simulink model "LOG_DATI_GPS_BMP_07_13_provacostanti"  (R2020b)
settings: Solver=ode4  StartTime=0.0  StopTime=Inf  FixedStep=0.02  RelTol=1e-3  EnableMultiTasking=on
PostLoadFcn:
  | , if any(exist('dsrtsu_mdlpostloadfcn', 'file') == [2, 3, 6]), try dsrtsu_mdlpostloadfcn('Execute', bdroot); catch fprintf('Error in PostLoadFcn (dsrtsu_mdlpostloadfcn) for model "%s":\n %s\n', bdroot, lasterr); end, end,
InitFcn:
  | , if any(exist('rtifpga_mdlclblib', 'file') ~= 0), rtifpga_mdlclblib('Init', bdroot); end,
values from neighbouring files (symbols this model uses):
  t_AP = 0.02    [AVVIO_YAK_DATA.m]
libraries: arduinolib x21, simulink_extras x6, svdutilitieslib x2, simulink x2
(part 1 of 3)
Description:
  | Standard RTI1006 template.
  | Supported MATLAB version:  R2020b.
settings Model: Tag=RTI1006  DSRTSU_INTERNAL_RTI_VER=570  DSRTSU_INTERNAL_RTI_TYPE=rti1006  RTICANMMDATA=struct('GeneralSetupData',struct('modelroot','C:\SUBTEAMS_2020_2021\SOFTWARE\AUTOPILOTA\drive1\Load_hardware\Arduino_v2_1','generalsettings',struct('filesettings',struct('destfolder',struct('Name','RTICANMM_FILES','Check',1),'buildfolder',struct('Name','.','Check',1),'AbsDestfolder',struct('Name','C:\SUBTEAMS_2020_2021\SOFTWARE\AUTOPILOTA\drive1\Load_hardware\Arduino_v2_1\RTICANMM_FILES'),'AbsBuildfolder',struct('Name','C:\SUBTEAMS_2020_2021\SOFTWARE\AUTOPILOTA\drive1\Load_hardware\Arduino_v2_1'))),'options',struct('addpaths',1,'rmpaths',1,'addtrcexclusion',true,'cannavigator',struct('checkmonitoring',0),'show_usrtrc',0,'use_usrtrc',0),'advanced',struct('options',ones(1,100)),'MPSetup',{{}},'RTI',struct('Type','ERT','Ver','','Date',''),'modelname','LOG_DATI_GPS_BMP_07_13_provacostanti','block','LOG_DATI_GPS_BMP_07_13_provacostanti'))  DSRTSU_INTERNAL_RTIFPGA=170  SILPILModeSetting=veronly  ExtModeTrigDuration=2  Creator=lapis-dspace  LastModifiedBy=lapis-dspace
settings DataIOCC: ReturnWorkspaceOutputs=off
settings OptimizationCC: BlockReduction=off  EnhancedBackFolding=on  PassReuseOutputArgsAs=Individual arguments  ZeroExternalMemoryAtStartup=off  ZeroInternalMemoryAtStartup=off  MaxStackSize=64  OptimizeBlockOrder=speed  DifferentSizesBufferReuse=on  OptimizationCustomize=off  EfficientTunableParamExpr=on
settings DebuggingCC: ParameterTunabilityLossMsg=error  PregeneratedLibrarySubsystemCodeDiagnostic=none  ArithmeticOperatorsInVariantConditions=warning
settings HardwareCC: ProdBitPerPointer=32  ProdBitPerSizeT=32  ProdBitPerPtrDiffT=32  ProdLargestAtomicInteger=Long  ProdLargestAtomicFloat=Double  ProdWordSize=32  ProdHWDeviceType=ARM Compatible->ARM Cortex  TargetIntDivRoundTo=Zero  TargetEndianess=LittleEndian  TargetHWDeviceType=Custom Processor->Custom
settings ModelReferenceCC: EnableParallelModelReferenceBuilds=on  ParallelModelReferenceMATLABWorkerInit=Load Top Model
settings SFSimCC: SimUseLocalCustomCode=off  MATLABDynamicMemAlloc=off  CustomCodeUndefinedFunction=UseInterfaceOnly
settings RTWCC: Description=Embedded Coder  SystemTargetFile=ert.tlc  HardwareBoard=Arduino Due  TemplateMakefile=ert_default_tmf  RTWUseLocalCustomCode=off  Toolchain=Arduino ARM  BuildConfiguration=Faster Runs
settings CodeAppCC: ForceParamTrailComments=on  IgnoreCustomStorageClasses=off  OperatorAnnotations=on  SimulinkDataObjDesc=on  SFDataObjDesc=on  InsertBlockDesc=on
settings ERTTargetCC: SupportContinuousTime=on  SupportVariableSizeSignals=on  ExtModeTransport=3  ExtModeStaticAllocSize=24576  ExtModeMexFile=ext_xcp  ExtModeIntrfLevel=Level2 - Open
settings ConfigComp: CovMetricSettings=dswe

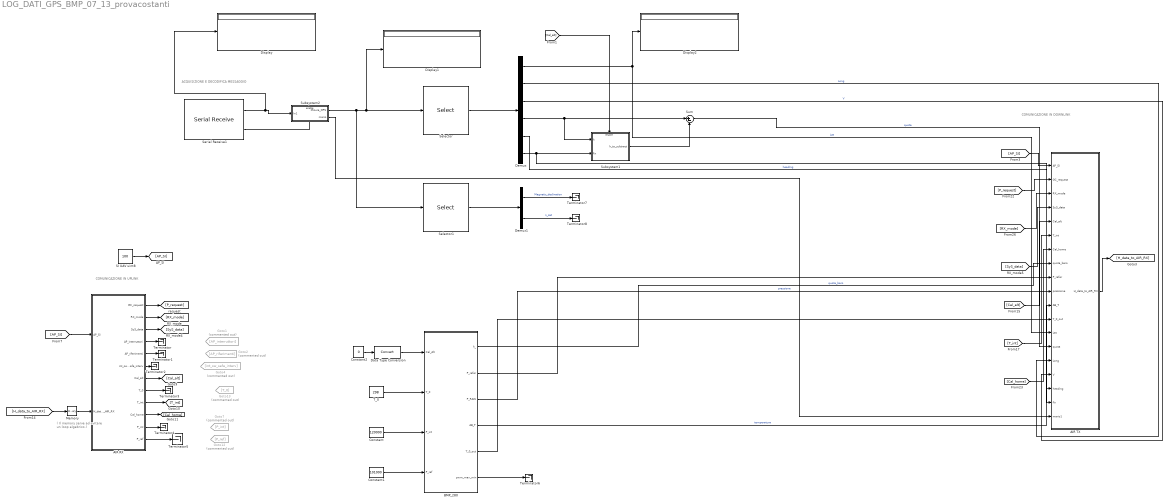
== system LOG_DATI_GPS_BMP_07_13_provacostanti ==
  note: ( Il memory serve ad evitare
      | un loop algebrico.)
  note: COMUNICAZIONE IN UPLINK
  note: COMUNICAZIONE IN DOWNLINK
  note: ACQUISIZIONE E DECODIFICA MESSAGGIO
  AIR RX : Subsystem
  AIR TX : Subsystem
  BMP_280 : Subsystem
  Constant : Constant  Value=120000
  Constant1 : Constant  Value=101000
  Constant2 : Constant  Value=0
  Data Type Conversion : DataTypeConversion
  Demux : Demux  Outputs=6
  Demux1 : Demux  Outputs=2
  Display : Display
  Display1 : Display
  Display2 : Display
  Goto1 : Goto  Commented=on  GotoTag=AP_interruttori
  Goto12 : Goto  Commented=on  GotoTag=P_ref
  Goto13 : Goto  Commented=on  GotoTag=T_0
  Goto2 : Goto  Commented=on  GotoTag=AP_riferimenti
  Goto4 : Goto  Commented=on  GotoTag=int_sw_safe_interv
  Goto7 : Goto  Commented=on  GotoTag=P_int
  Memory : Memory
  SI UAV uint8 : Constant  Value=100  OutDataTypeStr=uint8
  Selector : Selector  InputPortWidth=9  IndexOptions=Index vector (dialog)  Indices=[1 2 3 8 5 6]  OutputSizes=1
  Selector1 : Selector  InputPortWidth=9  IndexOptions=Index vector (dialog)  Indices=[4 7]  OutputSizes=1
  Serial Receive1 : arduinolib/Serial Receive  isARMArch=on  portNumber=1  DataType=uint8  Datalength=32  SampleTime=0.02  showOutStatus=on  blockPlatform=arduino
      settings: SourceProductBaseCode=ARDUINO
  Subsystem1 : Subsystem
  Subsystem2 : Subsystem
  Sum : Sum  Inputs=|+-
  T_0 : Constant  Value=298
  Terminator{,1..8} (9 alike) : Terminator
  wires:
  Constant/1 -> BMP_280/3(P_int)
  BMP_280/1(h_) -> AIR TX/8(quota_baro)  "quota_baro"
  T_0/1 -> BMP_280/2(T_0)
  BMP_280/3(P_RAW) -> AIR TX/10(pressione)  "pressione"
  BMP_280/5(T_0_out) -> AIR TX/12(T_0_out)
  BMP_280/2(P_refer) -> AIR TX/9(P_refer)
  BMP_280/6("pwm_max_min ") -> Terminator6/1
  Constant1/1 -> BMP_280/4(P_ref)
  Constant2/1 -> Data Type Conversion/1
  Data Type Conversion/1 -> BMP_280/1(Cal_Alt)
  AIR RX/9(T_int) -> [T_int]
  AIR RX/10(Cal_home) -> [Cal_home]
  AIR RX/8(T_0) -> Terminator3/1
  AIR RX/6(int_sw_safe_interv) -> Terminator2/1
  AIR RX/1(GC_request) -> [P_request]
  [AP_SI] -> AIR RX/1(AP_SI)
  AIR RX/12(P_ref) -> Terminator5/1
  [SyS_data] -> AIR TX/4(SyS_data)
  [Cal_home] -> AIR TX/7(Cal_home)
  [RX_mode] -> AIR TX/3(RX_mode)
  AIR RX/4(AP_interruttori) -> Terminator/1
  AIR RX/11(P_int) -> Terminator4/1
  [T_int] -> AIR TX/6(T_int)
  [H_data_to_AIR_RX] -> Memory/1
  AIR RX/5(AP_riferimenti) -> Terminator1/1
  [Cal_alt] -> AIR TX/5(Cal_alt)
  [P_request] -> AIR TX/2(GC_request)
  AIR RX/2(RX_mode) -> [RX_mode]
  Memory/1 -> AIR RX/2(H_data_to_AIR_RX)
  SI UAV uint8/1 -> [AP_SI]
  AIR RX/7(Cal_alt) -> [Cal_alt]
  AIR RX/3(SyS_data) -> [SyS_data]
  AIR TX/1(H_data_to_AIR_RX) -> [H_data_to_AIR_RX]
  [AP_SI] -> AIR TX/1(AP_SI)
  BMP_280/4(AB_T) -> AIR TX/11(AB_T)  "temperatura"
  Subsystem2/1(Misure_GPS) -> Selector1/1, Display1/1, Selector/1
  Demux/2 -> AIR TX/15(Long)  "Long"
  Demux1/1 -> Terminator7/1  "Magnetic_declination"
  Demux/6 -> AIR TX/18("fix "), Subsystem1/2(fix)
  Selector/1 -> Demux/1
  [Cal_alt] -> Subsystem1/Enable
  Demux/4 -> Sum/1, Subsystem1/1(h)
  Serial Receive1/1 -> Display/1, Subsystem2/1(In1)
  Demux1/2 -> Terminator8/1  "n_sat"
  Selector1/1 -> Demux1/1
  Demux/5 -> AIR TX/17(heading)  "heading"
  Demux/3 -> AIR TX/16(V)  "V"
  Demux/1 -> Display2/1, AIR TX/13(Lat)  "Lat"
  Sum/1 -> AIR TX/14(quota)  "quota"
  Subsystem2/2(mario) -> AIR TX/19(mario1)
  Subsystem1/1(h_to_subtract) -> Sum/2
  Serial Receive1/2 -> Subsystem2/Enable

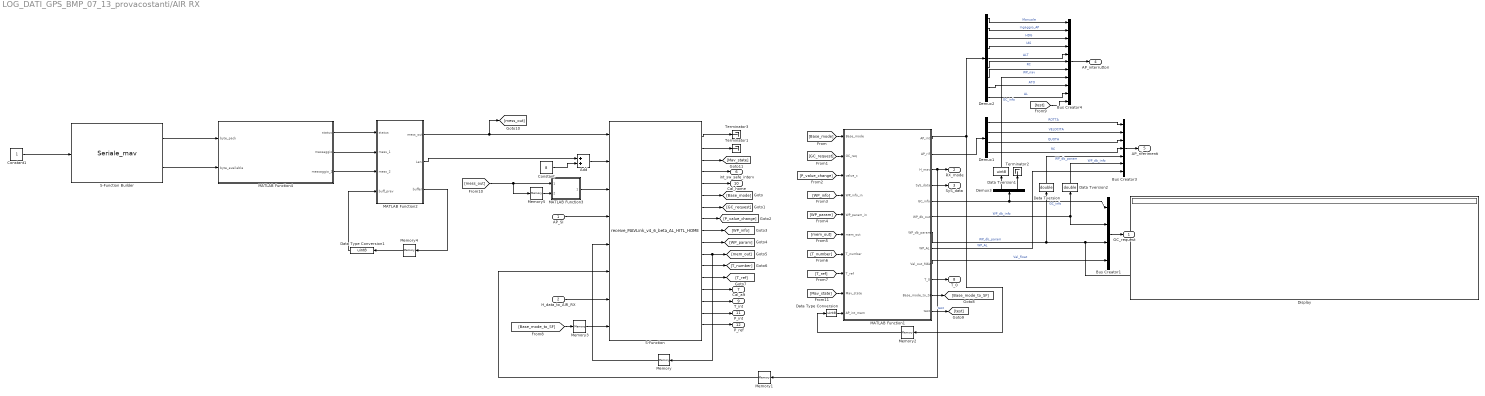
== system LOG_DATI_GPS_BMP_07_13_provacostanti/AIR RX ==
  AP_SI : Inport
  H_data_to_AIR_RX : Inport  Port=2
  Add : Sum  AccumDataTypeStr=int32
  Bus Creator1 : BusCreator  Inputs=4
  Bus Creator3 : BusCreator  Inputs=7
  Bus Creator4 : BusCreator  Inputs=11
  Constant : Constant  Value=8  OutDataTypeStr=int32  SampleTime=-1
  Constant1 : Constant  OutDataTypeStr=uint8
  Data Tversion : DataTypeConversion  OutDataTypeStr=double
  Data Tversion1 : DataTypeConversion  OutDataTypeStr=uint8
  Data Tversion2 : DataTypeConversion  OutDataTypeStr=double
  Data Type Conversion : DataTypeConversion  OutDataTypeStr=uint8
  Data Type Conversion1 : DataTypeConversion  OutDataTypeStr=uint8
  Demux1 : Demux
  Demux2 : Demux  Outputs=9
  Demux3 : Demux  Outputs=[1 2]
  Display : Display
      settings: Floating=on
  MATLAB Function1 : MATLAB Function  TreatAsAtomicUnit=on
  MATLAB Function2 : MATLAB Function  TreatAsAtomicUnit=on
  MATLAB Function3 : MATLAB Function  TreatAsAtomicUnit=on
  MATLAB Function4 : MATLAB Function  TreatAsAtomicUnit=on
  Memory : Memory  InheritSampleTime=on
  Memory1 : Memory  InheritSampleTime=on
  Memory2 : Memory  InitialCondition=[0 0 0 0 0 0 0 0 0]
  Memory3 : Memory
  Memory4 : Memory  InitialCondition=uint8(zeros(3,100))  InheritSampleTime=on
  Memory5 : Memory  InheritSampleTime=on
  S-Function : S-Function  FunctionName=receive_MAVLink_v4_6_beta_AL_HITL_HOME  SFunctionModules='receive_MAVLink_v4_6_beta_AL_HITL_HOME_wrapper'  SFunctionDeploymentMode=off  EnableBusSupport=off
  S-Function Builder : S-Function  InitFcn=try, set_param(gcb,'FunctionName','Seriale_mav'), end  FunctionName=Seriale_mav  SFunctionModules=Seriale_mav_wrapper  SFunctionDeploymentMode=off  EnableBusSupport=off  mask(S-Function Builder){}
      mask help: Simulink:masks:SFunctionBuilder_MD
      mask init:
      | val = [[.9  0.75 0.75 1 1 .9 .9 1]',[1 1 0.75 0.75 .9 .9 1 .9]'];try , sys = get_param(gcb,'SfunBuilderFcnName');if isempty(sys), sys = get_param(gcb,'FunctionName'); end,catch, sys = get_param(gcb,'FunctionName'); end
      settings: CopyFcn=set_param(gcbh,'LinkStatus','none')  PreSaveFcn=try, set_param(gcb,'FunctionName','Seriale_mav'), end  OpenFcn=sfunctionwizard(gcbh)
      mask Display: plot(val(:,1),val(:,2)),disp(sys),port_label('input',1,'inutile'),port_label('output',1,'Messaggio'),port_label('output',2,'serial_available')
  Terminator1 : Terminator
  Terminator2 : Terminator
  Terminator3 : Terminator
  GC_request : Outport  VectorParamsAs1DForOutWhenUnconnected=off
  RX_mode : Outport  Port=2  VectorParamsAs1DForOutWhenUnconnected=off
  SyS_data : Outport  Port=3  VectorParamsAs1DForOutWhenUnconnected=off
  AP_interruttori : Outport  Port=4  VectorParamsAs1DForOutWhenUnconnected=off
  AP_riferimenti : Outport  Port=5  VectorParamsAs1DForOutWhenUnconnected=off
  int_sw_safe_interv : Outport  Port=6  VectorParamsAs1DForOutWhenUnconnected=off
  Cal_alt : Outport  Port=7  VectorParamsAs1DForOutWhenUnconnected=off
  T_0 : Outport  Port=8  VectorParamsAs1DForOutWhenUnconnected=off
  T_int : Outport  Port=9  VectorParamsAs1DForOutWhenUnconnected=off
  Cal_home : Outport  Port=10  VectorParamsAs1DForOutWhenUnconnected=off
  P_int : Outport  Port=11  VectorParamsAs1DForOutWhenUnconnected=off
  P_ref : Outport  Port=12  VectorParamsAs1DForOutWhenUnconnected=off
  wires:
  H_data_to_AIR_RX/1 -> S-Function/7
  Memory1/1 -> S-Function/6
  Memory/1 -> S-Function/5
  Memory3/1 -> S-Function/8
  AP_SI/1 -> S-Function/4
  S-Function/5 -> Cal_home/1
  S-Function/4 -> int_sw_safe_interv/1
  S-Function/3 -> [Mav_state]
  S-Function/2 -> Terminator1/1
  S-Function/1 -> Terminator3/1
  S-Function/15 -> T_int/1
  S-Function/14 -> Cal_alt/1
  S-Function/13 -> [T_ref]
  S-Function/12 -> [T_number]
  S-Function/11 -> Memory/1, [mem_out]
  S-Function/10 -> [WP_param]
  S-Function/9 -> [WP_info]
  S-Function/8 -> [P_value_change]
  S-Function/6 -> [Base_mode]
  S-Function/7 -> [GC_request]
  Demux2/6 -> Bus Creator4/6  "RC"
  Data Tversion1/1 -> Bus Creator4/8  "GC_info"
  Memory2/1 -> Data Type Conversion/1
  Bus Creator1/1 -> GC_request/1
  Demux1/2 -> Bus Creator3/2  "VELOCITA"
  Demux2/5 -> Bus Creator4/5  "ALT"
  Demux2/1 -> Bus Creator4/1  "Manuale"
  Demux2/3 -> Bus Creator4/3  "HDG"
  [P_value_change] -> MATLAB Function1/3(value_c)
  Demux1/4 -> Bus Creator3/4  "RC"
  MATLAB Function1/2(AP_rif) -> Demux1/1
  Demux2/8 -> Bus Creator4/9  "ATO"
  MATLAB Function1/7(WP_db_param) -> Bus Creator1/3, Data Tversion/1  "WP_db_param"
  [GC_request] -> MATLAB Function1/2(GC_req)
  Demux2/2 -> Bus Creator4/2  "Ingaggio_AP"
  [mem_out] -> MATLAB Function1/6(mem_out)
  Bus Creator4/1 -> AP_interruttori/1
  MATLAB Function1/4(SyS_data) -> SyS_data/1
  MATLAB Function1/6(WP_db_out) -> Data Tversion2/1, Bus Creator1/2  "WP_db_info"
  [Mav_state] -> MATLAB Function1/9(Mav_state)
  Demux2/7 -> Bus Creator4/7  "WP_nav"
  [T_ref] -> MATLAB Function1/8(T_ref)
  Data Type Conversion/1 -> MATLAB Function1/10(AP_int_mem)
  Data Tversion2/1 -> Bus Creator3/6  "WP_db_info"
  Demux3/2 -> Terminator2/1
  [Base_mode] -> MATLAB Function1/1(Base_mode)
  [WP_param] -> MATLAB Function1/5(WP_param_in)
  Data Tversion/1 -> Bus Creator3/5  "WP_db_param"
  Demux3/1 -> Data Tversion1/1
  MATLAB Function1/3(H_mav) -> Memory1/1, RX_mode/1
  MATLAB Function1/9(Val_out_MAV) -> Bus Creator1/4  "Val_float"
  Bus Creator3/1 -> AP_riferimenti/1
  [T_number] -> MATLAB Function1/7(T_number)
  MATLAB Function1/5(GC_info) -> Demux3/1, Bus Creator1/1  "GC_info"
  MATLAB Function1/1(AP_int) -> Demux2/1, Memory2/1
  [WP_info] -> MATLAB Function1/4(WP_info_in)
  [Base_mode_to_SF] -> Memory3/1
  MATLAB Function1/11(Base_mode_to_SF) -> [Base_mode_to_SF]
  Demux1/3 -> Bus Creator3/3  "QUOTA"
  MATLAB Function1/12(test) -> [test]  "test"
  Demux2/4 -> Bus Creator4/4  "IAS"
  [test] -> Bus Creator4/11
  Demux1/1 -> Bus Creator3/1  "ROTTA"
  MATLAB Function1/8(WP_AL) -> Bus Creator3/7  "WP_AL"
  MATLAB Function1/10(T_0) -> T_0/1
  Demux2/9 -> Bus Creator4/10  "AL"
  MATLAB Function4/3(messaggio_2) -> MATLAB Function2/3(mess_2)
  MATLAB Function2/2(Len) -> Add/1
  MATLAB Function4/1(status) -> MATLAB Function2/1(status)
  MATLAB Function4/2(messaggio) -> MATLAB Function2/2(mess_1)
  Memory4/1 -> Data Type Conversion1/1
  MATLAB Function2/3(buffer) -> Memory4/1
  Constant/1 -> Add/2
  MATLAB Function2/1(mess_out) -> S-Function/1, [mess_out]
  MATLAB Function3/1(new_mex) -> S-Function/3
  Add/1 -> S-Function/2
  Data Type Conversion1/1 -> MATLAB Function2/4(buff_prev)
  Memory5/1 -> MATLAB Function3/2(mess_out_prev)
  [mess_out] -> Memory5/1, MATLAB Function3/1(mess_out)
  S-Function Builder/2 -> MATLAB Function4/2(byte_available)
  S-Function Builder/1 -> MATLAB Function4/1(byte_pack)
  Constant1/1 -> S-Function Builder/1
  S-Function/16 -> P_int/1
  S-Function/17 -> P_ref/1

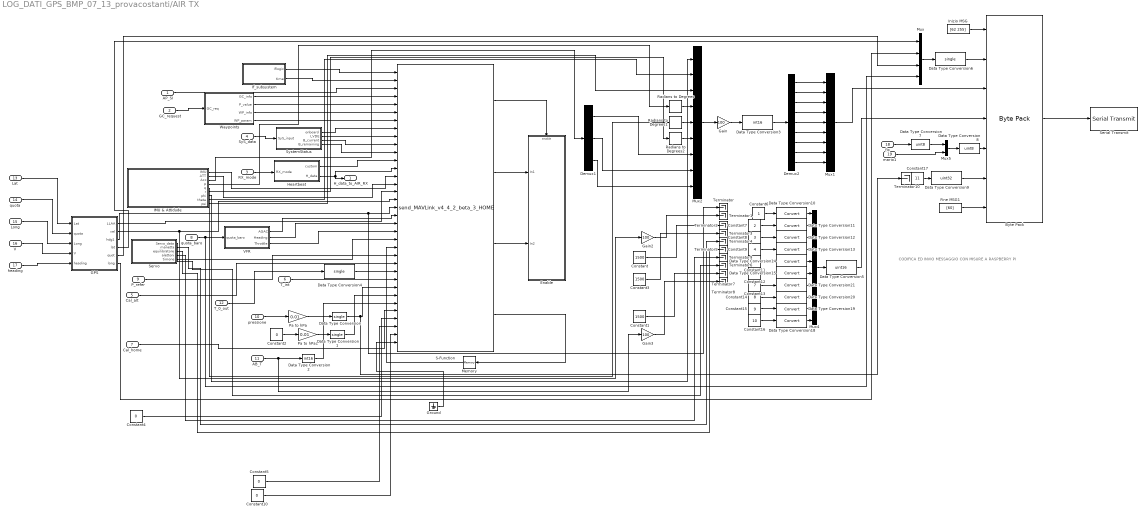
== system LOG_DATI_GPS_BMP_07_13_provacostanti/AIR TX ==
  note: CODIFICA ED INVIO MESSAGGIO CON MISURE A RASPBERRY PI
  AP_SI : Inport
  GC_request : Inport  Port=2
  RX_mode : Inport  Port=3
  SyS_data : Inport  Port=4
  Cal_alt : Inport  Port=5
  T_int : Inport  Port=6
  Cal_home : Inport  Port=7
  quota_baro : Inport  Port=8
  P_refer : Inport  Port=9
  pressione : Inport  Port=10
  AB_T : Inport  Port=11
  T_0_out : Inport  Port=12
  Lat : Inport  Port=13
  quota : Inport  Port=14
  Long : Inport  Port=15
  V : Inport  Port=16
  heading : Inport  Port=17
  "fix " : Inport  Port=18
  mario1 : Inport  Port=19
  Byte Pack : svdutilitieslib/Byte Pack  maskPackedDataType=uint8  datatypes={'uint8','single','int16','uint16','uint8','uint32','uint8'}  byteAlign=1  blockPlatform=arduinoert
      settings: SourceProductBaseCode=ANDROID,ARDUINO,ML_ARDUINO,ECCORTEXA,ECCORTEXR,SC_BEAGLEBONE_BLUE,EC_FREEDOM_BOARD,EC_FRDM_K64F,INTEL_BLOCKSET,JETSONCPU,MICROBIT,NUCLEO,NVIDIA,PX4AUTOPILOTS,RASPPIIO,STMICRODIS,TIC2000,XILINX_BLOCKSET
  Constant : Constant  Value=1500  OutDataTypeStr=double
  Constant1 : Constant  Value=1500  OutDataTypeStr=double
  Constant{2,4..5,10} (4 alike) : Constant  Value=0
  Constant11 : Constant  Value=5
  Constant12 : Constant  Value=6
  Constant13 : Constant  Value=7
  Constant14 : Constant  Value=8
  Constant15 : Constant  Value=9
  Constant16 : Constant  Value=10
  Constant17 : Constant  Value=11
  Constant3 : Constant  Value=1500  OutDataTypeStr=double
  Constant6 : Constant
  Constant7 : Constant  Value=2
  Constant8 : Constant  Value=3
  Constant9 : Constant  Value=4
  Data Type Conversion{,1,4,6} (4 alike) : DataTypeConversion  OutDataTypeStr=single
  Data Type Conversion{10..15,18..21} (10 alike) : DataTypeConversion
  Data Type Conversion2 : DataTypeConversion  OutDataTypeStr=int16
  Data Type Conversion3 : DataTypeConversion  OutDataTypeStr=int16
  Data Type Conversion5 : DataTypeConversion  OutDataTypeStr=uint16
  Data Type Conversion7 : DataTypeConversion  OutDataTypeStr=uint8
  Data Type Conversion8 : DataTypeConversion  OutDataTypeStr=uint8
  Data Type Conversion9 : DataTypeConversion  OutDataTypeStr=uint32
  Demux1 : Demux  Outputs=3
  Demux2 : Demux  Outputs=9
  "Enable " : Subsystem  TreatAsAtomicUnit=on
  Fine MSG1 : Constant  Value=[60]  OutDataTypeStr=uint8  SampleTime=t_AP
  GPS : Subsystem  SystemSampleTime=0.02
  Gain : Gain  Gain=100  OutDataTypeStr=single
  Gain2 : Gain  Gain=100
  Gain3 : Gain  Gain=100  OutDataTypeStr=double
  Ground : Ground
  Heartbeat : Subsystem  SystemSampleTime=1
  IMU & Attidude : Subsystem  SystemSampleTime=0.04
  If_subsystem : Subsystem
  Inizio MSG : Constant  Value=[62 255]  OutDataTypeStr=uint8  SampleTime=t_AP
  Memory : Memory
  Mux : Mux
  Mux1 : Mux  Inputs=9
  Mux2 : Mux  Inputs=9
  Mux4 : Mux  Inputs=10
  Mux5 : Mux  Inputs=2
  Pa to hPa : Gain  Gain=0.01
  Pa to hPa1 : Gain  Gain=0.01
  Radians to Degrees : simulink_extras/Transformations/Radians to Degrees
  Radians to Degrees1 : simulink_extras/Transformations/Radians to Degrees
  Radians to Degrees2 : simulink_extras/Transformations/Radians to Degrees
  S-Function : S-Function  FunctionName=send_MAVLink_v4_4_2_beta_3_HOME  SFunctionModules='send_MAVLink_v4_4_2_beta_3_HOME_wrapper'  SFunctionDeploymentMode=off  EnableBusSupport=off
  Serial Transmit : arduinolib/Serial Transmit  portNumber=0  sendmode=print  sendformat=Decimal  floatprecision=2  blockPlatform=arduino
  Servo : Subsystem  SystemSampleTime=0.5
  SystemStatus : Subsystem  SystemSampleTime=0.2
  Terminator{,1..10} (11 alike) : Terminator
  VFR : Subsystem  SystemSampleTime=0.5
  Waypoints : Subsystem  SystemSampleTime=1
  H_data_to_AIR_RX : Outport  VectorParamsAs1DForOutWhenUnconnected=off
  wires:
  If_subsystem/2(time) -> S-Function/2
  If_subsystem/1(iflogic) -> S-Function/1
  VFR/2(Heading) -> S-Function/20
  Heartbeat/2(H_data) -> H_data_to_AIR_RX/1, S-Function/13
  RX_mode/1 -> Heartbeat/1(RX_mode)
  S-Function/1 -> "Enable "/Enable
  AP_SI/1 -> S-Function/3
  Constant2/1 -> Pa to hPa1/1
  SyS_data/1 -> SystemStatus/1(SyS_input)
  S-Function/3 -> "Enable "/2(In2)
  SystemStatus/1(onboard) -> S-Function/8
  SystemStatus/4(B_remaining) -> S-Function/11
  T_int/1 -> S-Function/27
  SystemStatus/2(LVDE) -> S-Function/9
  Heartbeat/1(custom) -> S-Function/12
  Cal_alt/1 -> S-Function/25
  GC_request/1 -> Waypoints/1(GC_req)
  S-Function/4 -> Memory/1
  S-Function/2 -> "Enable "/1(In1)
  Waypoints/2(P_value) -> S-Function/5
  IMU & Attidude/2(ATT) -> S-Function/15
  Memory/1 -> S-Function/23
  Data Type Conversion1/1 -> S-Function/29
  Waypoints/1(GC_info) -> S-Function/4
  Servo/1(Servo_data) -> S-Function/22
  IMU & Attidude/1(IMU) -> S-Function/14
  Waypoints/3(WP_info) -> S-Function/6
  Pa to hPa1/1 -> Data Type Conversion1/1
  P_refer/1 -> S-Function/24
  GPS/1(LLAA) -> S-Function/16
  Data Type Conversion2/1 -> S-Function/30
  Constant10/1 -> S-Function/34
  SystemStatus/3(B_current) -> S-Function/10
  Cal_home/1 -> S-Function/31
  VFR/3(Throttle) -> S-Function/21
  Waypoints/4(WP_param) -> S-Function/7
  Constant4/1 -> S-Function/32
  VFR/1(AGAC) -> S-Function/19
  Constant5/1 -> S-Function/33
  Ground/1 -> S-Function/35
  pressione/1 -> Pa to hPa/1
  Pa to hPa/1 -> Data Type Conversion/1
  Data Type Conversion4/1 -> S-Function/26
  T_0_out/1 -> Data Type Conversion4/1
  Lat/1 -> GPS/1(Lat)
  quota/1 -> GPS/2(quota)
  Long/1 -> GPS/3(Long)
  V/1 -> GPS/4(V)
  heading/1 -> GPS/5(heading)
  GPS/4(lat) -> Mux/1
  mario1/1 -> Mux5/2
  Mux1/1 -> Byte Pack/3
  Demux2/3 -> Mux1/3
  Demux2/8 -> Mux1/8
  Servo/3(equilibratore) -> Terminator5/1
  Demux2/9 -> Mux1/9
  Mux2/1 -> Gain/1
  Data Type Conversion9/1 -> Byte Pack/6
  quota_baro/1 -> Mux/4, VFR/1(quota_baro)
  Demux2/7 -> Mux1/7
  IMU & Attidude/5(q) -> Radians to Degrees1/1
  Servo/4(alettoni) -> Terminator9/1
  Inizio MSG/1 -> Byte Pack/1
  GPS/3(hdg1) -> Terminator/1, S-Function/18
  Mux/1 -> Data Type Conversion6/1
  IMU & Attidude/7(phi) -> Mux2/1
  Demux2/1 -> Mux1/1
  Servo/5(timone) -> Terminator6/1
  Gain/1 -> Data Type Conversion3/1
  Data Type Conversion/1 -> Terminator10/1, S-Function/28
  Demux2/6 -> Mux1/6
  IMU & Attidude/9(psi) -> Mux2/3
  IMU & Attidude/6(r) -> Radians to Degrees2/1
  Radians to Degrees2/1 -> Mux2/6
  Data Type Conversion6/1 -> Byte Pack/2
  Fine MSG1/1 -> Byte Pack/7
  Gain2/1 -> Terminator1/1
  Demux2/4 -> Mux1/4
  Servo/2(manetta) -> Terminator4/1
  Data Type Conversion3/1 -> Demux2/1
  "fix "/1 -> Data Type Conversion7/1
  Demux1/3 -> Mux2/9
  GPS/5(quot) -> Mux/3
  Demux2/2 -> Mux1/2
  Demux1/1 -> Mux2/7
  Radians to Degrees/1 -> Mux2/4
  GPS/6(long) -> Mux/2
  AB_T/1 -> Gain3/1, Data Type Conversion2/1
  Mux5/1 -> Data Type Conversion8/1
  Data Type Conversion7/1 -> Mux5/1
  Radians to Degrees1/1 -> Mux2/5
  Demux1/2 -> Mux2/8
  IMU & Attidude/4(p) -> Radians to Degrees/1
  Demux2/5 -> Mux1/5
  Data Type Conversion8/1 -> Byte Pack/5
  GPS/2(vel) -> Gain2/1, S-Function/17
  Mux4/1 -> Data Type Conversion5/1
  IMU & Attidude/8(theta) -> Mux2/2
  IMU & Attidude/3(Acc) -> Demux1/1
  Constant/1 -> Terminator2/1
  Constant3/1 -> Terminator3/1
  Constant1/1 -> Terminator7/1
  Gain3/1 -> Terminator8/1
  Data Type Conversion10/1 -> Mux4/1
  Data Type Conversion11/1 -> Mux4/2
  Data Type Conversion12/1 -> Mux4/3
  Data Type Conversion13/1 -> Mux4/4
  Data Type Conversion14/1 -> Mux4/5
  Data Type Conversion15/1 -> Mux4/6
  Data Type Conversion21/1 -> Mux4/7
  Data Type Conversion20/1 -> Mux4/8
  Data Type Conversion19/1 -> Mux4/9
  Data Type Conversion18/1 -> Mux4/10
  Byte Pack/1 -> Serial Transmit/1
  Data Type Conversion5/1 -> Byte Pack/4
  Constant6/1 -> Data Type Conversion10/1
  Constant15/1 -> Data Type Conversion19/1
  Constant9/1 -> Data Type Conversion13/1
  Constant7/1 -> Data Type Conversion11/1
  Constant8/1 -> Data Type Conversion12/1
  Constant11/1 -> Data Type Conversion14/1
  Constant12/1 -> Data Type Conversion15/1
  Constant13/1 -> Data Type Conversion21/1
  Constant14/1 -> Data Type Conversion20/1
  Constant16/1 -> Data Type Conversion18/1
  Constant17/1 -> Data Type Conversion9/1

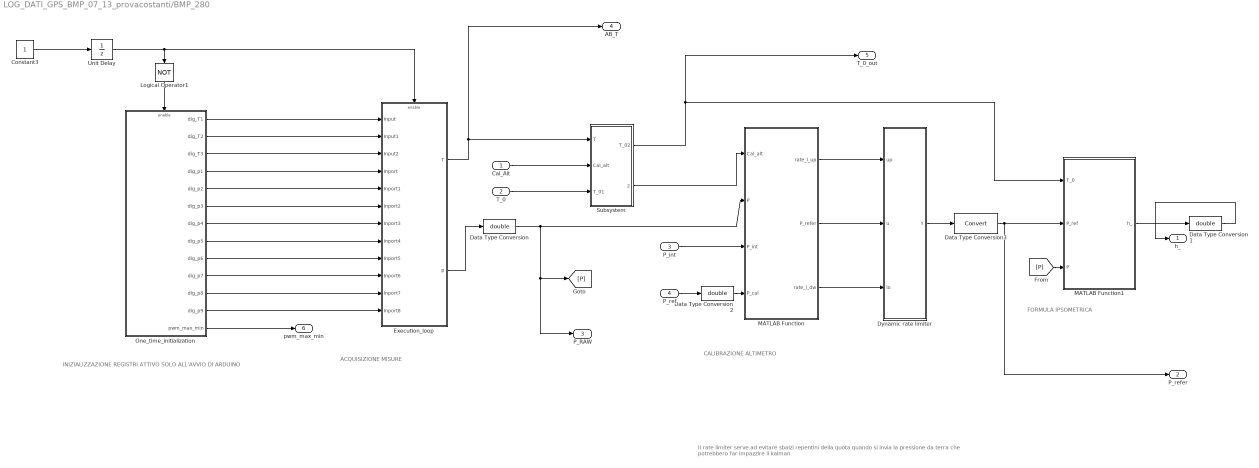
== system LOG_DATI_GPS_BMP_07_13_provacostanti/BMP_280 ==
  note: INIZIALIZZAZIONE REGISTRI
      | ATTIVO SOLO ALL'AVVIO DI ARDUINO
  note: Il rate limiter serve ad evitare sbalzi repentini della quota quando si invia la pressione da terra
      | che potrebbero far impazzire il kalman
  note: ACQUISIZIONE MISURE
  note: CALIBRAZIONE ALTIMETRO
  note: FORMULA IPSOMETRICA
  Cal_Alt : Inport
  T_0 : Inport  Port=2
  P_int : Inport  Port=3
  P_ref : Inport  Port=4
  Constant3 : Constant  OutDataTypeStr=boolean  SampleTime=t_AP
  Data Type Conversion : DataTypeConversion  OutDataTypeStr=double
  Data Type Conversion1 : DataTypeConversion  OutDataTypeStr=double
  Data Type Conversion2 : DataTypeConversion  OutDataTypeStr=double
  Data Type Conversion3 : DataTypeConversion
  Dynamic rate limiter : Subsystem
  Execution_loop : Subsystem  TreatAsAtomicUnit=on
  Logical Operator1 : Logic  Operator=NOT  AllPortsSameDT=off  OutDataTypeStr=boolean
  MATLAB Function : MATLAB Function  TreatAsAtomicUnit=on
  MATLAB Function1 : MATLAB Function  TreatAsAtomicUnit=on
  One_time_initialization : Subsystem  TreatAsAtomicUnit=on
  Subsystem : Subsystem
  Unit Delay : UnitDelay  SampleTime=-1  HasFrameUpgradeWarning=on
  h_ : Outport  VectorParamsAs1DForOutWhenUnconnected=off
  P_refer : Outport  Port=2  VectorParamsAs1DForOutWhenUnconnected=off
  P_RAW : Outport  Port=3  VectorParamsAs1DForOutWhenUnconnected=off
  AB_T : Outport  Port=4  VectorParamsAs1DForOutWhenUnconnected=off
  T_0_out : Outport  Port=5  VectorParamsAs1DForOutWhenUnconnected=off
  "pwm_max_min " : Outport  Port=6  VectorParamsAs1DForOutWhenUnconnected=off
  wires:
  One_time_initialization/11(dig_p8) -> Execution_loop/11(Inport7)
  One_time_initialization/4(dig_p1) -> Execution_loop/4(Inport)
  One_time_initialization/7(dig_p4) -> Execution_loop/7(Inport3)
  Execution_loop/2(p) -> Data Type Conversion/1
  Unit Delay/1 -> Execution_loop/Enable, Logical Operator1/1
  One_time_initialization/12(dig_p9) -> Execution_loop/12(Inport8)
  One_time_initialization/9(dig_p6) -> Execution_loop/9(Inport5)
  One_time_initialization/2(dig_T2) -> Execution_loop/2(Input1)
  One_time_initialization/6(dig_p3) -> Execution_loop/6(Inport2)
  One_time_initialization/10(dig_p7) -> Execution_loop/10(Inport6)
  Logical Operator1/1 -> One_time_initialization/Enable
  One_time_initialization/5(dig_p2) -> Execution_loop/5(Inport1)
  One_time_initialization/3(dig_T3) -> Execution_loop/3(Input2)
  One_time_initialization/1(dig_T1) -> Execution_loop/1(Input)
  Constant3/1 -> Unit Delay/1
  Data Type Conversion/1 -> [P], P_RAW/1, MATLAB Function/2(P)
  One_time_initialization/8(dig_p5) -> Execution_loop/8(Inport4)
  MATLAB Function1/1(h_) -> Data Type Conversion1/1
  Data Type Conversion1/1 -> h_/1
  Execution_loop/1(T) -> AB_T/1, Subsystem/1(T)
  Cal_Alt/1 -> Subsystem/2(Cal_alt)
  Subsystem/2(Cal_alt2) -> MATLAB Function/1(Cal_alt)
  Subsystem/1(T_02) -> MATLAB Function1/1(T_0), T_0_out/1
  T_0/1 -> Subsystem/3(T_01)
  One_time_initialization/13(pwm_max_min) -> "pwm_max_min "/1
  MATLAB Function/2(P_refer) -> Dynamic rate limiter/2(u)
  P_int/1 -> MATLAB Function/3(P_int)
  P_ref/1 -> Data Type Conversion2/1
  MATLAB Function/3(rate_l_dw) -> Dynamic rate limiter/3(lo)
  MATLAB Function/1(rate_l_up) -> Dynamic rate limiter/1(up)
  [P] -> MATLAB Function1/3(P)
  Data Type Conversion2/1 -> MATLAB Function/4(P_cal)
  Dynamic rate limiter/1(Y) -> Data Type Conversion3/1
  Data Type Conversion3/1 -> P_refer/1, MATLAB Function1/2(P_ref)

== system LOG_DATI_GPS_BMP_07_13_provacostanti/Subsystem1 ==
  h : Inport
  fix : Inport  Port=2
  Enable : EnablePort
  Constant : Constant
  Constant1 : Constant  Value=2
  Constant2 : Constant  Value=0
  Constant3 : Constant  Value=3
  Equal : RelationalOperator  Operator===  OutDataTypeStr=boolean  RndMeth=Simplest
  Equal1 : RelationalOperator  Operator===  OutDataTypeStr=boolean  RndMeth=Simplest
  Equal2 : RelationalOperator  Operator===  OutDataTypeStr=boolean  RndMeth=Simplest
  OR : Logic  Operator=OR  Inputs=3  IconShape=distinctive  AllPortsSameDT=off  OutDataTypeStr=boolean
  Switch : Switch  Criteria=u2 > Threshold
  h_to_subtract : Outport  VectorParamsAs1DForOutWhenUnconnected=off
  wires:
  Constant/1 -> Equal/2
  Equal/1 -> OR/1
  Constant1/1 -> Equal1/2
  Equal1/1 -> OR/2
  h/1 -> Switch/1
  OR/1 -> Switch/2
  Constant2/1 -> Switch/3
  Switch/1 -> h_to_subtract/1
  Equal2/1 -> OR/3
  Constant3/1 -> Equal2/2
  fix/1 -> Equal2/1, Equal1/1, Equal/1

== system LOG_DATI_GPS_BMP_07_13_provacostanti/Subsystem2 ==
  In1 : Inport
  Enable : EnablePort
  Create_message : MATLAB Function  TreatAsAtomicUnit=on
  Subsystem : Subsystem
  Misure_GPS : Outport  VectorParamsAs1DForOutWhenUnconnected=off
  mario : Outport  Port=2  VectorParamsAs1DForOutWhenUnconnected=off
  wires:
  In1/1 -> Create_message/1(byte_pack)
  Create_message/2(messaggio) -> Subsystem/1(In1)
  Create_message/1(status) -> Subsystem/Enable
  Subsystem/1(Outport) -> Misure_GPS/1
  Subsystem/2(mario) -> mario/1

== system LOG_DATI_GPS_BMP_07_13_provacostanti/AIR TX/Enable  ==
  In1 : Inport
  In2 : Inport  Port=2
  Enable : EnablePort
  Chart : Stateflow chart  TreatAsAtomicUnit=on
  wires:
  In2/1 -> Chart/2(Len)
  In1/1 -> Chart/1(datain)

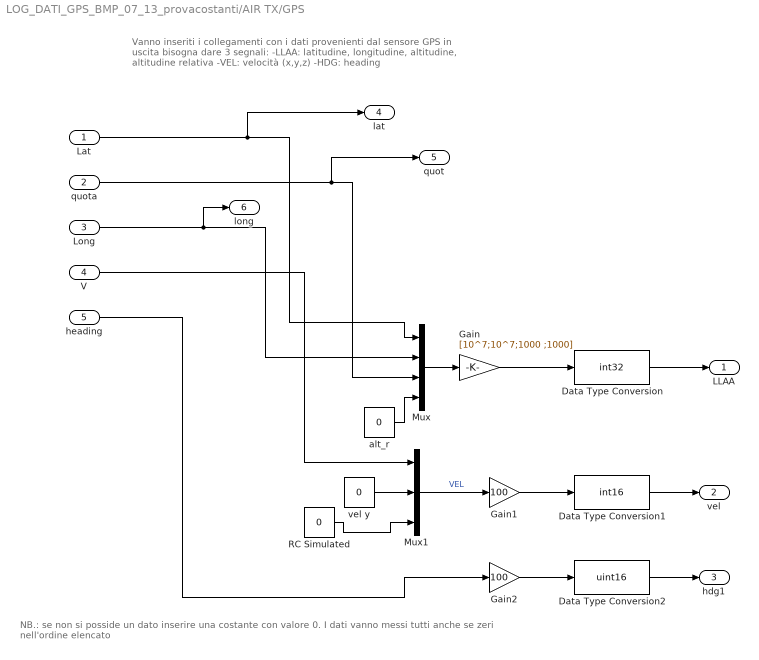
== system LOG_DATI_GPS_BMP_07_13_provacostanti/AIR TX/GPS ==
  note: NB.: se non si posside un dato inserire una costante con valore 0. I dati vanno messi tutti anche se zeri nell'ordine elencato
  note: Vanno inseriti i collegamenti con i dati provenienti dal sensore GPS
      | in uscita bisogna dare 3 segnali:
      |
      | -LLAA: latitudine, longitudine, altitudine, altitudine relativa
      | -VEL: velocità (x,y,z)
      | -HDG: heading
  Lat : Inport
  quota : Inport  Port=2
  Long : Inport  Port=3
  V : Inport  Port=4
  heading : Inport  Port=5
  Data Type Conversion : DataTypeConversion  OutDataTypeStr=int32  RndMeth=Simplest
  Data Type Conversion1 : DataTypeConversion  OutDataTypeStr=int16  RndMeth=Simplest
  Data Type Conversion2 : DataTypeConversion  OutDataTypeStr=uint16  RndMeth=Simplest
  Gain : Gain  Gain=[10^7;10^7;1000 ;1000]
  Gain1 : Gain  Gain=100
  Gain2 : Gain  Gain=100
  Mux : Mux
  Mux1 : Mux  Inputs=3
  RC Simulated : Constant  Value=0
  alt_r : Constant  Value=0
  vel y : Constant  Value=0  OutDataTypeStr=double
  LLAA : Outport  VectorParamsAs1DForOutWhenUnconnected=off
  vel : Outport  Port=2  VectorParamsAs1DForOutWhenUnconnected=off
  hdg1 : Outport  Port=3  VectorParamsAs1DForOutWhenUnconnected=off
  lat : Outport  Port=4
  quot : Outport  Port=5
  long : Outport  Port=6
  wires:
  quota/1 -> quot/1, Mux/3
  Gain2/1 -> Data Type Conversion2/1
  Data Type Conversion/1 -> LLAA/1
  Gain/1 -> Data Type Conversion/1
  Data Type Conversion1/1 -> vel/1
  Long/1 -> long/1, Mux/2
  Lat/1 -> lat/1, Mux/1
  RC Simulated/1 -> Mux1/3
  vel y/1 -> Mux1/2
  heading/1 -> Gain2/1
  Mux/1 -> Gain/1
  V/1 -> Mux1/1
  Mux1/1 -> Gain1/1  "VEL"
  Data Type Conversion2/1 -> hdg1/1
  alt_r/1 -> Mux/4
  Gain1/1 -> Data Type Conversion1/1

== system LOG_DATI_GPS_BMP_07_13_provacostanti/AIR TX/Heartbeat ==
  note: Vanno inseriti i collegamenti con i dati provenienti dalla ricezione (stazione di terra) e gli allarmi
      | in uscita bisogna dare 2 vettori costituiti da:
      | -I:
      | -custom code (su può mettere ciò che si vuole)
      | -II:
      | -vettore di 2 componenti: tido di veivolo e tipo di autopilota
      | -vettore di due componenti che è creato tramite la matlabfuncition
  RX_mode : Inport
  Alarm set : MATLAB Function  TreatAsAtomicUnit=on
  Constant : Constant  Value=0
  Constant1 : Constant  Value=[0 0]
  Data Type Conversion : DataTypeConversion  OutDataTypeStr=uint32
  Data Type Conversion1 : DataTypeConversion  OutDataTypeStr=uint8
  Mux : Mux  Inputs=2
  Type fixed_wing Autopilot generic : Constant  Value=[1;0]  OutDataTypeStr=uint8
  custom : Outport  VectorParamsAs1DForOutWhenUnconnected=off
  H_data : Outport  Port=2  VectorParamsAs1DForOutWhenUnconnected=off
  wires:
  Constant/1 -> Data Type Conversion/1
  Data Type Conversion1/1 -> H_data/1
  Data Type Conversion/1 -> custom/1
  RX_mode/1 -> Alarm set/2(Rx_mode)
  Constant1/1 -> Alarm set/1(Alarm)
  Type fixed_wing Autopilot generic/1 -> Mux/1
  Alarm set/1(H_mav) -> Mux/2
  Mux/1 -> Data Type Conversion1/1

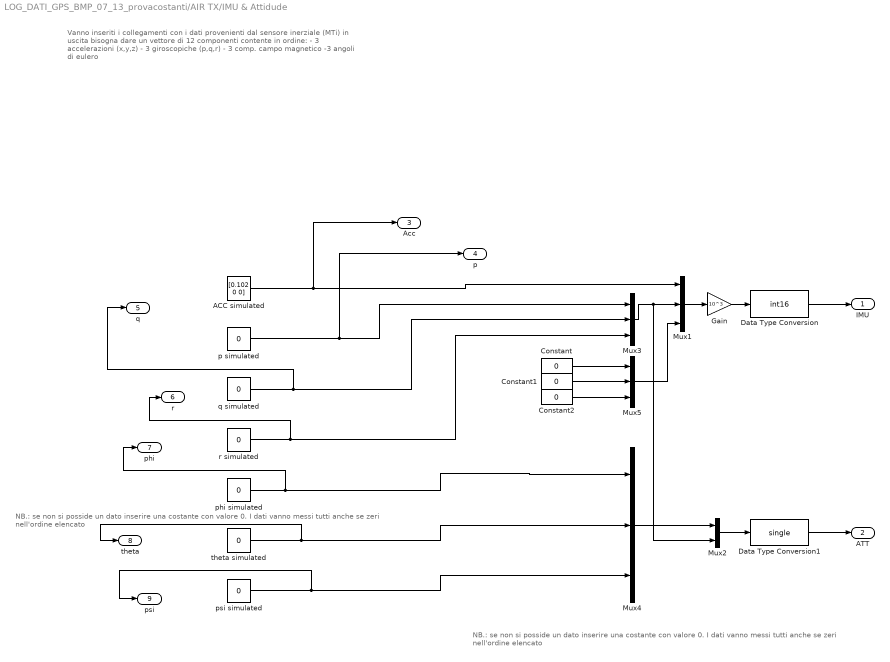
== system LOG_DATI_GPS_BMP_07_13_provacostanti/AIR TX/IMU & Attidude ==
  note: NB.: se non si posside un dato inserire una costante con valore 0. I dati vanno messi tutti anche se zeri nell'ordine elencato
  note: Vanno inseriti i collegamenti con i dati provenienti dal sensore inerziale (MTi)
      | in uscita bisogna dare un vettore di 12 componenti contente in ordine:
      | - 3 accelerazioni (x,y,z)
      | - 3 giroscopiche (p,q,r)
      | - 3 comp. campo magnetico
      | -3 angoli di eulero
  note: NB.: se non si posside un dato inserire una costante con valore 0. I dati vanno messi tutti anche se zeri nell'ordine elencato
  ACC simulated : Constant  Value=[0.102 0 0]
  Constant : Constant  Value=0  OutDataTypeStr=double  SampleTime=0.02
  Constant1 : Constant  Value=0  OutDataTypeStr=double  SampleTime=0.02
  Constant2 : Constant  Value=0  OutDataTypeStr=double  SampleTime=0.02
  Data Type Conversion : DataTypeConversion  OutDataTypeStr=int16  RndMeth=Simplest
  Data Type Conversion1 : DataTypeConversion  OutDataTypeStr=single
  Gain : Gain  Gain=10^3
  Mux{1,3..5} (4 alike) : Mux  Inputs=3
  Mux2 : Mux  Inputs=2
  p simulated : Constant  Value=0
  phi simulated : Constant  Value=0
  psi simulated : Constant  Value=0
  q simulated : Constant  Value=0
  r simulated : Constant  Value=0
  theta simulated : Constant  Value=0
  IMU : Outport  VectorParamsAs1DForOutWhenUnconnected=off
  ATT : Outport  Port=2  VectorParamsAs1DForOutWhenUnconnected=off
  Acc : Outport  Port=3
  p : Outport  Port=4
  q : Outport  Port=5
  r : Outport  Port=6
  phi : Outport  Port=7
  theta : Outport  Port=8
  psi : Outport  Port=9
  wires:
  r simulated/1 -> r/1, Mux3/3
  q simulated/1 -> q/1, Mux3/2
  psi simulated/1 -> psi/1, Mux4/3
  Constant1/1 -> Mux5/2
  Gain/1 -> Data Type Conversion/1
  Mux2/1 -> Data Type Conversion1/1
  Data Type Conversion/1 -> IMU/1
  Data Type Conversion1/1 -> ATT/1
  Mux4/1 -> Mux2/1
  Constant/1 -> Mux5/1
  Constant2/1 -> Mux5/3
  Mux5/1 -> Mux1/3
  Mux3/1 -> Mux1/2, Mux2/2
  phi simulated/1 -> phi/1, Mux4/1
  p simulated/1 -> p/1, Mux3/1
  Mux1/1 -> Gain/1
  ACC simulated/1 -> Acc/1, Mux1/1
  theta simulated/1 -> theta/1, Mux4/2

== system LOG_DATI_GPS_BMP_07_13_provacostanti/AIR TX/If_subsystem ==
  note: Blocco per la temporizzazione dell'invio dei messaggi
  Data Type Conversion3 : DataTypeConversion  OutDataTypeStr=uint32  RndMeth=Simplest
  Gain : Gain  Gain=100
  Subsystem : Subsystem
  iflogic_function : MATLAB Function  TreatAsAtomicUnit=on
  iflogic : Outport  VectorParamsAs1DForOutWhenUnconnected=off
  time : Outport  Port=2  VectorParamsAs1DForOutWhenUnconnected=off
  wires:
  Subsystem/3(time) -> Gain/1
  Subsystem/2(H_10) -> iflogic_function/2(H10)
  Subsystem/1(H_50) -> iflogic_function/1(H50)
  Gain/1 -> Data Type Conversion3/1
  Data Type Conversion3/1 -> time/1
  iflogic_function/1(iflogic) -> iflogic/1

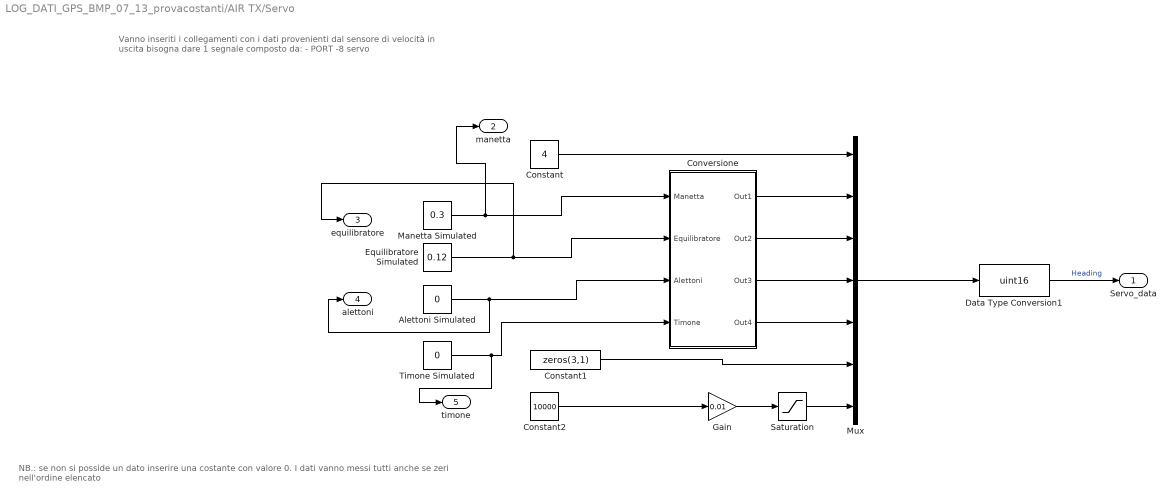
== system LOG_DATI_GPS_BMP_07_13_provacostanti/AIR TX/Servo ==
  note: NB.: se non si posside un dato inserire una costante con valore 0. I dati vanno messi tutti anche se zeri nell'ordine elencato
  note: Vanno inseriti i collegamenti con i dati provenienti dal sensore di velocità
      | in uscita bisogna dare 1 segnale composto da:
      |
      | -  PORT
      | -8 servo
  Alettoni Simulated : Constant  Value=0
  Constant : Constant  Value=4
  Constant1 : Constant  Value=zeros(3,1)
  Constant2 : Constant  Value=10000
  Conversione : Subsystem
  Data Type Conversion1 : DataTypeConversion  OutDataTypeStr=uint16  RndMeth=Simplest
  Equilibratore Simulated : Constant  Value=0.12
  Gain : Gain  Gain=0.01
  Manetta Simulated : Constant  Value=0.3
  Mux : Mux  Inputs=7
  Saturation : Saturate  UpperLimit=4000  LowerLimit=0
  Timone Simulated : Constant  Value=0
  Servo_data : Outport  VectorParamsAs1DForOutWhenUnconnected=off
  manetta : Outport  Port=2
  equilibratore : Outport  Port=3
  alettoni : Outport  Port=4
  timone : Outport  Port=5
  wires:
  Constant2/1 -> Gain/1
  Equilibratore Simulated/1 -> equilibratore/1, Conversione/2(Equilibratore)
  Alettoni Simulated/1 -> alettoni/1, Conversione/3(Alettoni)
  Timone Simulated/1 -> timone/1, Conversione/4(Timone)
  Manetta Simulated/1 -> manetta/1, Conversione/1(Manetta)
  Conversione/3(Out3) -> Mux/4
  Constant1/1 -> Mux/6
  Conversione/1(Out1) -> Mux/2
  Mux/1 -> Data Type Conversion1/1
  Constant/1 -> Mux/1
  Data Type Conversion1/1 -> Servo_data/1  "Heading"
  Conversione/4(Out4) -> Mux/5
  Saturation/1 -> Mux/7
  Gain/1 -> Saturation/1
  Conversione/2(Out2) -> Mux/3

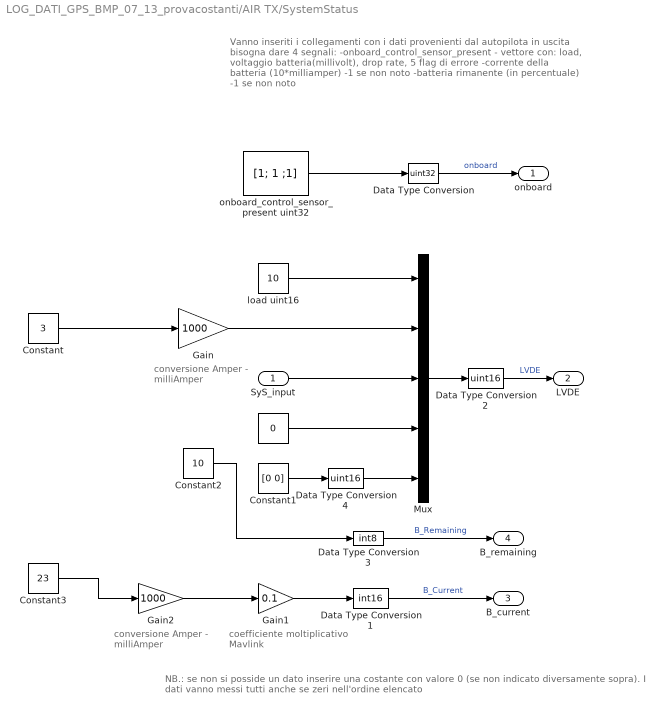
== system LOG_DATI_GPS_BMP_07_13_provacostanti/AIR TX/SystemStatus ==
  note: coefficiente moltiplicativo Mavlink
  note: conversione
      | Amper - milliAmper
  note: NB.: se non si posside un dato inserire una costante con valore 0 (se non indicato diversamente sopra).
      | I dati vanno messi tutti anche se zeri nell'ordine elencato
  note: Vanno inseriti i collegamenti con i dati provenienti dal autopilota
      | in uscita bisogna dare 4 segnali:
      |
      | -onboard_control_sensor_present
      | - vettore con: load, voltaggio batteria(millivolt), drop rate, 5 flag di errore
      | -corrente della batteria (10*milliamper) -1 se non noto
      | -batteria rimanente (in percentuale) -1 se non noto
  note: conversione
      | Amper - milliAmper
  SyS_input : Inport
  " " : Constant  Value=0  OutDataTypeStr=uint16
  Constant : Constant  Value=3
  Constant1 : Constant  Value=[0 0]
  Constant2 : Constant  Value=10
  Constant3 : Constant  Value=23
  Data Type Conversion : DataTypeConversion  OutDataTypeStr=uint32
  Data Type Conversion1 : DataTypeConversion  OutDataTypeStr=int16
  Data Type Conversion2 : DataTypeConversion  OutDataTypeStr=uint16
  Data Type Conversion3 : DataTypeConversion  OutDataTypeStr=int8
  Data Type Conversion4 : DataTypeConversion  OutDataTypeStr=uint16
  Gain : Gain  Gain=1000  OutDataTypeStr=uint16
  Gain1 : Gain  Gain=0.1  OutDataTypeStr=int16
  Gain2 : Gain  Gain=1000  OutDataTypeStr=int16
  Mux : Mux  Inputs=5
  load uint16 : Constant  Value=10  OutDataTypeStr=uint16
  onboard_control_sensor_present uint32 : Constant  Value=[1; 1 ;1]  OutDataTypeStr=uint32
  onboard : Outport  VectorParamsAs1DForOutWhenUnconnected=off
  LVDE : Outport  Port=2  VectorParamsAs1DForOutWhenUnconnected=off
  B_current : Outport  Port=3  VectorParamsAs1DForOutWhenUnconnected=off
  B_remaining : Outport  Port=4  VectorParamsAs1DForOutWhenUnconnected=off
  wires:
  Gain2/1 -> Gain1/1
  Gain1/1 -> Data Type Conversion1/1
  " "/1 -> Mux/4
  Data Type Conversion4/1 -> Mux/5
  Constant1/1 -> Data Type Conversion4/1
  SyS_input/1 -> Mux/3
  Data Type Conversion3/1 -> B_remaining/1  "B_Remaining"
  Data Type Conversion1/1 -> B_current/1  "B_Current"
  Data Type Conversion2/1 -> LVDE/1  "LVDE"
  Data Type Conversion/1 -> onboard/1  "onboard"
  Mux/1 -> Data Type Conversion2/1
  Gain/1 -> Mux/2
  load uint16/1 -> Mux/1
  onboard_control_sensor_present uint32/1 -> Data Type Conversion/1
  Constant/1 -> Gain/1
  Constant2/1 -> Data Type Conversion3/1
  Constant3/1 -> Gain2/1

== system LOG_DATI_GPS_BMP_07_13_provacostanti/AIR TX/VFR ==
  note: NB.: se non si posside un dato inserire una costante con valore 0. I dati vanno messi tutti anche se zeri nell'ordine elencato
  note: Vanno inseriti i collegamenti con i dati provenienti dal sensore di velocità
      | in uscita bisogna dare 3 segnali:
      |
      | -  AGAC: airspeed, groundspeed,altitudine, rateo salita
      | -Heading
      | -Throttle: spinta o rpm del motore
  note: inserire 100/massimo valore
      | deve uscire una percentuale
      | FISSATO PER QUOTA IL 5-5-2016
  quota_baro : Inport
  " Heading simulated" : Constant  Value=50
  Data Type Conversion3 : DataTypeConversion  OutDataTypeStr=single
  Data Type Conversion4 : DataTypeConversion  OutDataTypeStr=int16
  Data Type Conversion5 : DataTypeConversion  OutDataTypeStr=uint16
  Mux : Mux
  RC simulated : Constant  Value=0
  Rpm simulated : Constant  Value=1000
  TAS simulated : Constant  Value=20
  v simulated : Constant  Value=20
  AGAC : Outport
  Heading : Outport  Port=2
  Throttle : Outport  Port=3
  wires:
  TAS simulated/1 -> Mux/1
  RC simulated/1 -> Mux/4
  Data Type Conversion5/1 -> Throttle/1
  Data Type Conversion4/1 -> Heading/1
  " Heading simulated"/1 -> Data Type Conversion4/1
  quota_baro/1 -> Mux/3
  Mux/1 -> Data Type Conversion3/1
  Data Type Conversion3/1 -> AGAC/1
  v simulated/1 -> Mux/2
  Rpm simulated/1 -> Data Type Conversion5/1

== system LOG_DATI_GPS_BMP_07_13_provacostanti/AIR TX/Waypoints ==
  GC_req : Inport
  Bus Selector3 : BusSelector  OutputSignals=Val_float,WP_db_info,WP_db_param,GC_info
  MATLAB Function : MATLAB Function  TreatAsAtomicUnit=on
  GC_info : Outport  VectorParamsAs1DForOutWhenUnconnected=off
  P_value : Outport  Port=2  VectorParamsAs1DForOutWhenUnconnected=off
  WP_info : Outport  Port=3  VectorParamsAs1DForOutWhenUnconnected=off
  WP_param : Outport  Port=4  VectorParamsAs1DForOutWhenUnconnected=off
  wires:
  Bus Selector3/1 -> P_value/1  "<Val_float>"
  MATLAB Function/2(WP_param) -> WP_param/1
  Bus Selector3/3 -> MATLAB Function/2(WP_param_in)  "<WP_db_param>"
  MATLAB Function/1(WP_info) -> WP_info/1
  Bus Selector3/2 -> MATLAB Function/1(WP_info_in)  "<WP_db_info>"
  Bus Selector3/4 -> MATLAB Function/3(GC_info), GC_info/1  "<GC_info>"
  GC_req/1 -> Bus Selector3/1

== system LOG_DATI_GPS_BMP_07_13_provacostanti/BMP_280/Dynamic rate limiter ==
  note: U(k)
  note: Y(k)
  up : Inport
  u : Inport  Port=2
  lo : Inport  Port=3
  Delay Input2 : UnitDelay  Description=Store in Global RAM  DisableCoverage=on  InitialCondition=101325  SampleTime=-1  HasFrameUpgradeWarning=on
  Difference Inputs1 : Sum  Description=Add in CPU  DisableCoverage=on  Inputs=+-  OutDataTypeStr=Inherit: Inherit via back propagation
  Difference Inputs2 : Sum  Description=Add in CPU  OutDataTypeStr=Inherit: Inherit via back propagation
  FixPt Data Type Duplicate : DataTypeDuplicate  DisableCoverage=on  NumInputPorts=7
  Saturation Dynamic : simulink/Discontinuities/Saturation Dynamic  OutMin=[]  OutMax=[]  OutDataTypeStr=Inherit: Same as second input  OutDataType=fixdt(1, 16)  OutScaling=2^-10  DoSatur=off
  delta fall limit : Product  DisableCoverage=on  Inputs=**  OutDataTypeStr=Inherit: Inherit via back propagation  SaturateOnIntegerOverflow=on
  delta rise limit : Product  DisableCoverage=on  Inputs=**  OutDataTypeStr=Inherit: Inherit via back propagation  SaturateOnIntegerOverflow=on
  sample time : SampleTimeMath  DisableCoverage=on  TsampMathOp=Ts Only  weightValue=1
  Y : Outport  InitialOutput=0  VectorParamsAs1DForOutWhenUnconnected=off
  wires:
  delta rise limit/1 -> FixPt Data Type Duplicate/6, Saturation Dynamic/1
  Difference Inputs2/1 -> Y/1, Delay Input2/1, FixPt Data Type Duplicate/1
  up/1 -> delta rise limit/1
  Saturation Dynamic/1 -> Difference Inputs2/1, FixPt Data Type Duplicate/7
  Delay Input2/1 -> Difference Inputs1/2, FixPt Data Type Duplicate/2, Difference Inputs2/2  "Y(k-1)"
  Difference Inputs1/1 -> FixPt Data Type Duplicate/4, Saturation Dynamic/2  "( U(k) - Y(k-1) )"
  u/1 -> Difference Inputs1/1, FixPt Data Type Duplicate/5, sample time/1
  lo/1 -> delta fall limit/1
  sample time/1 -> delta fall limit/2, delta rise limit/2
  delta fall limit/1 -> FixPt Data Type Duplicate/3, Saturation Dynamic/3

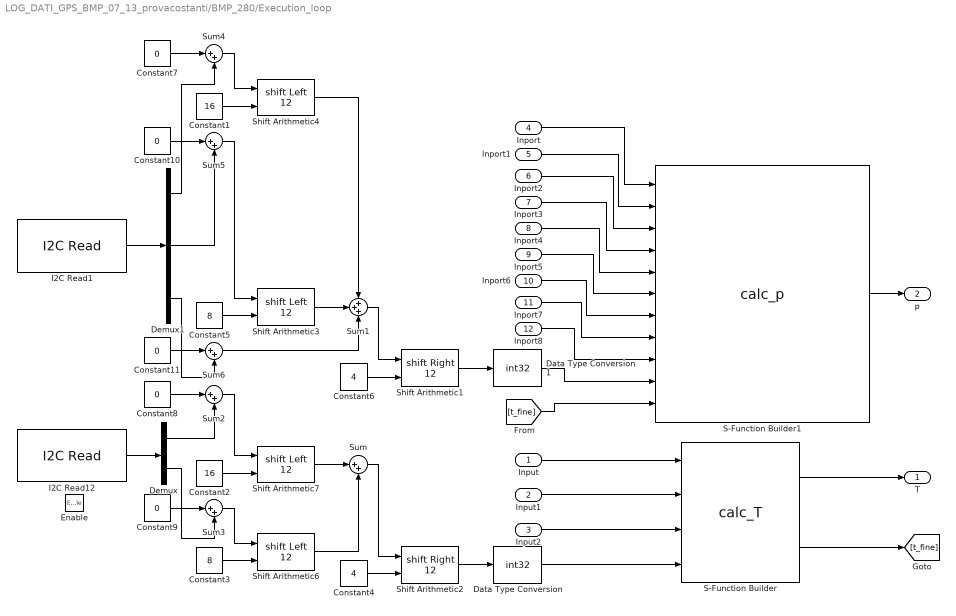
== system LOG_DATI_GPS_BMP_07_13_provacostanti/BMP_280/Execution_loop ==
  Input : Inport
  Input1 : Inport  Port=2
  Input2 : Inport  Port=3
  Inport : Inport  Port=4
  Inport1 : Inport  Port=5
  Inport2 : Inport  Port=6
  Inport3 : Inport  Port=7
  Inport4 : Inport  Port=8
  Inport5 : Inport  Port=9
  Inport6 : Inport  Port=10
  Inport7 : Inport  Port=11
  Inport8 : Inport  Port=12
  Enable : EnablePort
  Constant1 : Constant  Value=16
  Constant{7..11} (5 alike) : Constant  Value=0  OutDataTypeStr=uint32
  Constant2 : Constant  Value=16
  Constant3 : Constant  Value=8
  Constant4 : Constant  Value=4
  Constant5 : Constant  Value=8
  Constant6 : Constant  Value=4
  Data Type Conversion : DataTypeConversion  OutDataTypeStr=int32
  Data Type Conversion1 : DataTypeConversion  OutDataTypeStr=int32
  Demux : Demux  Outputs=2
  Demux1 : Demux  Outputs=3
  I2C Read1 : arduinolib/I2C Read  Priority=2  I2CModule=0  Mode=Master  SlaveAddress=hex2dec( '76' )  SlaveByteOrder=BigEndian  Direction=Receiver  RegisterAddressMode=on  RegisterAddress=hex2dec( 'F7' )  SlaveDataType=uint8  DataLength=3  NoAck=off  RepeatedStart=off  OutputStatus=off  blockPlatform=arduino  SampleTime=t_AP
      settings: AttributesFormatString=Priority=%<Priority>  SourceProductBaseCode=ARDUINO
  I2C Read12 : arduinolib/I2C Read  Priority=1  I2CModule=0  Mode=Master  SlaveAddress=hex2dec( '76' )  SlaveByteOrder=BigEndian  Direction=Receiver  RegisterAddressMode=on  RegisterAddress=hex2dec( 'FA' )  SlaveDataType=uint8  DataLength=2  NoAck=off  RepeatedStart=off  OutputStatus=off  blockPlatform=arduino  SampleTime=t_AP
      settings: AttributesFormatString=Priority=%<Priority>  SourceProductBaseCode=ARDUINO
  S-Function Builder : S-Function  InitFcn=try, set_param(gcb,'FunctionName','calc_T'), end  FunctionName=calc_T  SFunctionModules=calc_T_wrapper  SFunctionDeploymentMode=off  EnableBusSupport=off  mask(S-Function Builder){}
      mask help: Simulink:masks:SFunctionBuilder_MD
      mask init: same as LOG_DATI_GPS_BMP_07_13_provacostanti/AIR RX/S-Function Builder
      settings: CopyFcn=set_param(gcbh,'LinkStatus','none')  PreSaveFcn=try, set_param(gcb,'FunctionName','calc_T'), end  OpenFcn=sfunctionwizard(gcbh)
      mask Display: plot(val(:,1),val(:,2)),disp(sys),port_label('input',1,'dig_T1'),port_label('input',2,'dig_T2'),port_label('input',3,'dig_T3'),port_label('input',4,'adc_T'),port_label('output',1,'T'),port_label('output',2,'t_fine')
  S-Function Builder1 : S-Function  InitFcn=try, set_param(gcb,'FunctionName','calc_p'), end  FunctionName=calc_p  SFunctionModules=calc_p_wrapper  SFunctionDeploymentMode=off  EnableBusSupport=off  mask(S-Function Builder){}
      mask help: Simulink:masks:SFunctionBuilder_MD
      mask init: same as LOG_DATI_GPS_BMP_07_13_provacostanti/AIR RX/S-Function Builder
      settings: CopyFcn=set_param(gcbh,'LinkStatus','none')  PreSaveFcn=try, set_param(gcb,'FunctionName','calc_p'), end  OpenFcn=sfunctionwizard(gcbh)
      mask Display: plot(val(:,1),val(:,2)),disp(sys),port_label('input',1,'dig_p1'),port_label('input',2,'dig_p2'),port_label('input',3,'dig_p3'),port_label('input',4,'dig_p4'),port_label('input',5,'dig_p5'),port_label('input',6,'dig_p6'),port_label('input',7,'dig_p7'),port_label('input',8,'dig_p8'),port_label('input',9,'dig_p9'),port_label('input',10,'adc_P'),port_label('input',11,'t_fine'),port_label('output',1,'p')
  Shift Arithmetic1 : ArithShift  BitShiftNumberSource=Input port  BitShiftNumber=12  BitShiftDirection=Right
      settings: InputPortMap=u0,p1
  Shift Arithmetic2 : ArithShift  BitShiftNumberSource=Input port  BitShiftNumber=12  BitShiftDirection=Right
      settings: InputPortMap=u0,p1
  Shift Arithmetic{3..4,6..7} (4 alike) : ArithShift  BitShiftNumberSource=Input port  BitShiftNumber=12  BitShiftDirection=Left
      settings: InputPortMap=u0,p1
  Sum{,2..6} (6 alike) : Sum  Inputs=|++
  Sum1 : Sum  Inputs=+++
  T : Outport  VectorParamsAs1DForOutWhenUnconnected=off
  p : Outport  Port=2  VectorParamsAs1DForOutWhenUnconnected=off
  wires:
  Inport6/1 -> S-Function Builder1/7
  Demux1/1 -> Sum4/2
  I2C Read1/1 -> Demux1/1
  Demux/1 -> Sum2/2
  I2C Read12/1 -> Demux/1
  [t_fine] -> S-Function Builder1/11
  S-Function Builder/2 -> [t_fine]
  Inport8/1 -> S-Function Builder1/9
  Inport7/1 -> S-Function Builder1/8
  Inport5/1 -> S-Function Builder1/6
  Inport4/1 -> S-Function Builder1/5
  Inport3/1 -> S-Function Builder1/4
  Inport2/1 -> S-Function Builder1/3
  Inport1/1 -> S-Function Builder1/2
  Inport/1 -> S-Function Builder1/1
  Data Type Conversion1/1 -> S-Function Builder1/10
  Sum6/1 -> Sum1/3
  Demux1/3 -> Sum6/2
  Constant11/1 -> Sum6/1
  Sum4/1 -> Shift Arithmetic4/1
  Shift Arithmetic3/1 -> Sum1/2
  Demux1/2 -> Sum5/2
  Constant10/1 -> Sum5/1
  Sum5/1 -> Shift Arithmetic3/1
  S-Function Builder1/1 -> p/1
  Constant7/1 -> Sum4/1
  Sum1/1 -> Shift Arithmetic1/1
  Constant6/1 -> Shift Arithmetic1/2
  Constant1/1 -> Shift Arithmetic4/2
  Shift Arithmetic1/1 -> Data Type Conversion1/1
  Constant5/1 -> Shift Arithmetic3/2
  Shift Arithmetic4/1 -> Sum1/1
  Data Type Conversion/1 -> S-Function Builder/4
  Sum3/1 -> Shift Arithmetic6/1
  Demux/2 -> Sum3/2
  Constant9/1 -> Sum3/1
  Constant8/1 -> Sum2/1
  Sum2/1 -> Shift Arithmetic7/1
  Sum/1 -> Shift Arithmetic2/1
  Shift Arithmetic6/1 -> Sum/2
  Shift Arithmetic7/1 -> Sum/1
  Constant2/1 -> Shift Arithmetic7/2
  Constant3/1 -> Shift Arithmetic6/2
  Input/1 -> S-Function Builder/1
  Input1/1 -> S-Function Builder/2
  Input2/1 -> S-Function Builder/3
  S-Function Builder/1 -> T/1
  Constant4/1 -> Shift Arithmetic2/2
  Shift Arithmetic2/1 -> Data Type Conversion/1
